simulink model "Motor_CD_Controlador_Paralelo"  (R2020b)
settings: Solver=VariableStepAuto  StartTime=0.0  StopTime=10.0  RelTol=1e-3
values from neighbouring files (symbols this model uses):
  Ki = 9.6    [WorkSpace.mat]
  Kp = 0.813559322034    [WorkSpace.mat]
libraries: cstblocks x1
settings Model: Creator=danielcastro  LastModifiedBy=danielcastro

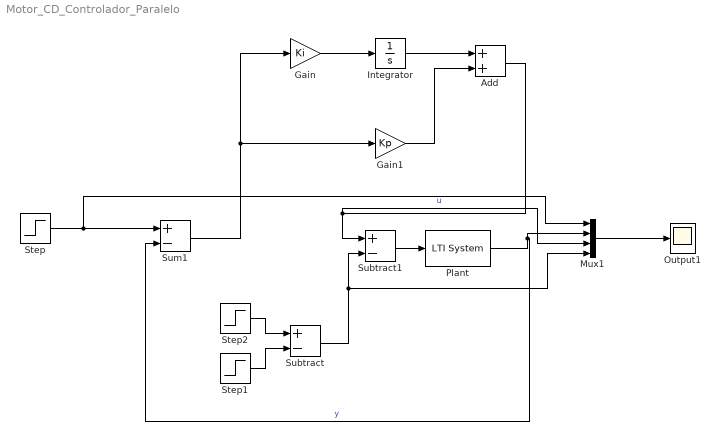
== system Motor_CD_Controlador_Paralelo ==
  Add : Sum
  Gain : Gain  Gain=Ki
  Gain1 : Gain  Gain=Kp
  Integrator : Integrator
  Mux1 : Mux
  Output1 : Scope
  Plant : cstblocks/LTI System  sys=G  IC=[]
  Step : Step  Time=0.1  After=4  SampleTime=0
  Step1 : Step  Time=1.2  SampleTime=0
  Step2 : Step  Time=0.7  SampleTime=0
  Subtract : Sum  Inputs=+-
  Subtract1 : Sum  Inputs=+-
  Sum1 : Sum  Inputs=+-
  wires:
  Gain1/1 -> Add/2
  Integrator/1 -> Add/1
  Gain/1 -> Integrator/1
  Subtract1/1 -> Plant/1
  Plant/1 -> Mux1/2, Sum1/2  "y"
  Step/1 -> Mux1/1, Sum1/1
  Step1/1 -> Subtract/2
  Sum1/1 -> Gain/1, Gain1/1
  Mux1/1 -> Output1/1
  Step2/1 -> Subtract/1
  Add/1 -> Subtract1/1, Mux1/3  "u"
  Subtract/1 -> Mux1/4, Subtract1/2
